simulink model "amila"  (R2013a)
settings: Solver=VariableStepDiscrete  SolverMode=SingleTasking  StartTime=0.0  StopTime=5000  RelTol=1e-3
undefined symbols (not defined in the file or in its folder): gcbh, sfp, xlBlockLoadCallback
libraries: xbsIndex_r4 x4681, dspsigops x32, xps_library x30, casper_library_misc x27, casper_library_delays x2
(part 4 of 43)

== system amila/chan1 ==
  fft_shift : Inport
  sync : Inport  Port=2
  din : Inport  Port=3
  Convert8 : xbsIndex_r4/Convert  gui_display_data_type=Boolean  arith_type=Boolean  n_bits=3  bin_pt=0  float_type=Single  exp_bits=8  fraction_bits=24  quantization=Truncate  overflow=Wrap  en=off  latency=0  dbl_ovrd=off  pipeline=off  block_type=convert
      settings: block_version=11.4
  Logical1 : xbsIndex_r4/Logical  logical_function=OR  inputs=4  en=off  latency=1  precision=Full  arith_type=Unsigned  n_bits=16  bin_pt=0  align_bp=on  dbl_ovrd=off  block_type=logical
  Subsystem6 : Subsystem
  a0p0_1st_shift1 : Subsystem  mask{shift=1, latency=0}
      mask prompts: shift "Number bits to shift right by"; latency "Shift latency"
  bus_create5 : Subsystem  AncestorBlock=casper_library_flow_control/bus_create  mask(bus_create){inputNum=8}
      mask prompts: inputNum "Number of inputs:"
      mask init:
      | bus_create_init(gcb,...
      |     'inputNum', inputNum);
  bus_expand : Subsystem  AncestorBlock=casper_library_flow_control/bus_expand  mask(bus_expand){mode=divisions of equal size, outputNum=4, outputWidth=1, outputBinaryPt=0, outputArithmeticType=0, show_format=off, outputToWorkspace=off, variablePrefix=out, outputToModelAsWell=on}
      mask prompts: outputNum "Number of outputs:"; outputWidth "Output width:"; outputBinaryPt "Output binary point position:"; outputArithmeticType "Output arithmetic type (ufix=0, fix=1, bool=2):"; show_format "Print format string?"; outputToWorkspace "Output to workspace?"; variablePrefix "Variable name prefix:"; outputToModelAsWell "Output to model as well?"
      mask help:
      | Expands a 'bus' made using a bus_create or Xilinx
      | concat block.
      | The input will be divided into the specified number
      | of outputs with the specified arithmetic types.
      | Divisions are made from most significant bit.
      mask init: same as amila/bus_expand6
      settings: AttributesFormatString=4 outputs
      mask TypeOptions mode: divisions of equal size | divisions of arbitrary size
      mask Callback mode: bus_expand_callback();
      mask Callback outputWidth: bus_expand_callback();
      mask Callback outputToWorkspace: bus_expand_callback();
  fft_core : xbsIndex_r4/Black Box  init_code=fft_core2_config  sim_method=Inactive  verbose=off  block_type=blackbox2
  unbus0_2 : Subsystem  AncestorBlock=casper_library_flow_control/bus_expand  mask(bus_expand){mode=divisions of equal size, outputNum=16, outputWidth=18, outputBinaryPt=17, outputArithmeticType=1, show_format=off, outputToWorkspace=off, variablePrefix=out, outputToModelAsWell=on}
      mask prompts: outputNum "Number of outputs:"; outputWidth "Output width:"; outputBinaryPt "Output binary point position:"; outputArithmeticType "Output arithmetic type (ufix=0, fix=1, bool=2):"; show_format "Print format string?"; outputToWorkspace "Output to workspace?"; variablePrefix "Variable name prefix:"; outputToModelAsWell "Output to model as well?"
      mask help:
      | Expands a 'bus' made using a bus_create or Xilinx
      | concat block.
      | The input will be divided into the specified number
      | of outputs with the specified arithmetic types.
      | Divisions are made from most significant bit.
      mask init: same as amila/bus_expand6
      settings: AttributesFormatString=16 outputs
      mask TypeOptions mode: divisions of equal size | divisions of arbitrary size
      mask Callback mode: bus_expand_callback();
      mask Callback outputWidth: bus_expand_callback();
      mask Callback outputToWorkspace: bus_expand_callback();
  sync_out : Outport
  dout : Outport  Port=2
  fft_of : Outport  Port=3
  wires:
  unbus0_2/10(out7) -> Subsystem6/11(In10)
  unbus0_2/12(out5) -> Subsystem6/13(In12)
  unbus0_2/3(out14) -> Subsystem6/4(In3)
  unbus0_2/6(out11) -> Subsystem6/7(In6)
  unbus0_2/16(lsb_out1) -> Subsystem6/17(In16)
  unbus0_2/14(out3) -> Subsystem6/15(In14)
  unbus0_2/5(out12) -> Subsystem6/6(In5)
  unbus0_2/15(out2) -> Subsystem6/16(In15)
  unbus0_2/11(out6) -> Subsystem6/12(In11)
  unbus0_2/9(out8) -> Subsystem6/10(In9)
  unbus0_2/1(msb_out16) -> Subsystem6/2(In1)
  unbus0_2/13(out4) -> Subsystem6/14(In13)
  unbus0_2/2(out15) -> Subsystem6/3(In2)
  unbus0_2/7(out10) -> Subsystem6/8(In7)
  unbus0_2/8(out9) -> Subsystem6/9(In8)
  unbus0_2/4(out13) -> Subsystem6/5(In4)
  sync/1 -> Subsystem6/1(sync)
  bus_create5/1(bus_out) -> dout/1
  fft_shift/1 -> fft_core/1
  a0p0_1st_shift1/1(sync_out) -> fft_core/2
  a0p0_1st_shift1/2(dout1) -> fft_core/3
  a0p0_1st_shift1/3(dout2) -> fft_core/4
  a0p0_1st_shift1/4(dout3) -> fft_core/5
  a0p0_1st_shift1/5(dout4) -> fft_core/6
  a0p0_1st_shift1/6(dout5) -> fft_core/7
  a0p0_1st_shift1/8(dout7) -> fft_core/9
  a0p0_1st_shift1/9(dout8) -> fft_core/10
  a0p0_1st_shift1/10(dout9) -> fft_core/11
  a0p0_1st_shift1/11(dout10) -> fft_core/12
  a0p0_1st_shift1/12(dout11) -> fft_core/13
  a0p0_1st_shift1/13(dout12) -> fft_core/14
  a0p0_1st_shift1/14(dout13) -> fft_core/15
  a0p0_1st_shift1/15(dout14) -> fft_core/16
  a0p0_1st_shift1/16(dout15) -> fft_core/17
  a0p0_1st_shift1/17(dout16) -> fft_core/18
  din/1 -> unbus0_2/1(bus_in)
  Subsystem6/8(Out7) -> a0p0_1st_shift1/8(din7)
  Subsystem6/13(Out12) -> a0p0_1st_shift1/13(din12)
  Subsystem6/11(Out10) -> a0p0_1st_shift1/11(din10)
  Subsystem6/16(Out15) -> a0p0_1st_shift1/16(din15)
  Subsystem6/14(Out13) -> a0p0_1st_shift1/14(din13)
  Subsystem6/10(Out9) -> a0p0_1st_shift1/10(din9)
  Subsystem6/6(Out5) -> a0p0_1st_shift1/6(din5)
  Subsystem6/7(Out6) -> a0p0_1st_shift1/7(din6)
  Subsystem6/2(Out1) -> a0p0_1st_shift1/2(din1)
  Subsystem6/3(Out2) -> a0p0_1st_shift1/3(din2)
  Subsystem6/9(Out8) -> a0p0_1st_shift1/9(din8)
  Subsystem6/1(sync_out) -> a0p0_1st_shift1/1(sync_in)
  Subsystem6/12(Out11) -> a0p0_1st_shift1/12(din11)
  Subsystem6/15(Out14) -> a0p0_1st_shift1/15(din14)
  Subsystem6/17(Out16) -> a0p0_1st_shift1/17(din16)
  Subsystem6/4(Out3) -> a0p0_1st_shift1/4(din3)
  Subsystem6/5(Out4) -> a0p0_1st_shift1/5(din4)
  a0p0_1st_shift1/7(dout6) -> fft_core/8
  bus_expand/3(out2) -> Logical1/3
  bus_expand/2(out3) -> Logical1/2
  bus_expand/4(lsb_out1) -> Logical1/4
  bus_expand/1(msb_out4) -> Logical1/1
  Logical1/1 -> Convert8/1
  Convert8/1 -> fft_of/1
  fft_core/1 -> sync_out/1
  fft_core/5 -> bus_create5/4(in4)
  fft_core/7 -> bus_create5/6(in6)
  fft_core/3 -> bus_create5/2(in2)
  fft_core/4 -> bus_create5/3(in3)
  fft_core/9 -> bus_create5/8(in8)
  fft_core/8 -> bus_create5/7(in7)
  fft_core/2 -> bus_create5/1(in1)
  fft_core/6 -> bus_create5/5(in5)
  fft_core/10 -> bus_expand/1(bus_in)

== system amila/clk_frequency ==
  reg_out : Inport
  amila_clk_frequency_user_data_in : xbsIndex_r4/Gateway Out  inherit_from_input=off  hdl_port=on  timing_constraint=None  locs_specified=off  LOCs={}  UseAsDAC=off  DACChannel='1'  block_type=gatewayout
  convert : xbsIndex_r4/Convert  gui_display_data_type=Fixed-point  arith_type=Unsigned  n_bits=32  bin_pt=0  float_type=Single  exp_bits=8  fraction_bits=24  quantization=Truncate  overflow=Wrap  en=off  latency=0  dbl_ovrd=off  pipeline=off  block_type=convert
  sim_reg_out : Outport
  wires:
  amila_clk_frequency_user_data_in/1 -> sim_reg_out/1
  convert/1 -> amila_clk_frequency_user_data_in/1
  reg_out/1 -> convert/1

== system amila/ct_tvg ==
  note: This TVG should result in each packet containing
      | its frequeny value every 16 bits
      | (assuming the ct is working properly)
  enable : Inport
  sync_in : Inport  Port=2
  din : Inport  Port=3
  Concat{1..4} (4 alike) : xbsIndex_r4/Concat  num_inputs=2  dbl_ovrd=off  block_type=concat
  Concat5 : xbsIndex_r4/Concat  num_inputs=4  dbl_ovrd=off  block_type=concat
  Convert{,1..7} (8 alike) : xbsIndex_r4/Convert  gui_display_data_type=Fixed-point  arith_type=Unsigned  n_bits=channel_bits*2  bin_pt=0  float_type=Single  exp_bits=8  fraction_bits=24  quantization=Truncate  overflow=Wrap  en=off  latency=0  dbl_ovrd=off  pipeline=off  block_type=convert
      settings: block_version=11.4
  Counter1 : xbsIndex_r4/Counter  cnt_type=Free Running  cnt_to=10  operation=Up  start_count=2  cnt_by_val=8  arith_type=Unsigned  n_bits=num_channels_bits  bin_pt=0  load_pin=off  rst=on  en=off  explicit_period=on  period=1  dbl_ovrd=off  use_behavioral_HDL=off  implementation=Fabric  block_type=counter
      settings: block_version=11.4
  Counter2 : xbsIndex_r4/Counter  cnt_type=Free Running  cnt_to=10  operation=Up  start_count=0  cnt_by_val=8  arith_type=Unsigned  n_bits=num_channels_bits  bin_pt=0  load_pin=off  rst=on  en=off  explicit_period=on  period=1  dbl_ovrd=off  use_behavioral_HDL=off  implementation=Fabric  block_type=counter
      settings: block_version=11.4
  Counter3 : xbsIndex_r4/Counter  cnt_type=Free Running  cnt_to=10  operation=Up  start_count=3  cnt_by_val=8  arith_type=Unsigned  n_bits=num_channels_bits  bin_pt=0  load_pin=off  rst=on  en=off  explicit_period=on  period=1  dbl_ovrd=off  use_behavioral_HDL=off  implementation=Fabric  block_type=counter
      settings: block_version=11.4
  Counter4 : xbsIndex_r4/Counter  cnt_type=Free Running  cnt_to=10  operation=Up  start_count=1  cnt_by_val=8  arith_type=Unsigned  n_bits=num_channels_bits  bin_pt=0  load_pin=off  rst=on  en=off  explicit_period=on  period=1  dbl_ovrd=off  use_behavioral_HDL=off  implementation=Fabric  block_type=counter
      settings: block_version=11.4
  Counter5 : xbsIndex_r4/Counter  cnt_type=Free Running  cnt_to=10  operation=Up  start_count=6  cnt_by_val=8  arith_type=Unsigned  n_bits=num_channels_bits  bin_pt=0  load_pin=off  rst=on  en=off  explicit_period=on  period=1  dbl_ovrd=off  use_behavioral_HDL=off  implementation=Fabric  block_type=counter
      settings: block_version=11.4
  Counter6 : xbsIndex_r4/Counter  cnt_type=Free Running  cnt_to=10  operation=Up  start_count=4  cnt_by_val=8  arith_type=Unsigned  n_bits=num_channels_bits  bin_pt=0  load_pin=off  rst=on  en=off  explicit_period=on  period=1  dbl_ovrd=off  use_behavioral_HDL=off  implementation=Fabric  block_type=counter
      settings: block_version=11.4
  Counter7 : xbsIndex_r4/Counter  cnt_type=Free Running  cnt_to=10  operation=Up  start_count=7  cnt_by_val=8  arith_type=Unsigned  n_bits=num_channels_bits  bin_pt=0  load_pin=off  rst=on  en=off  explicit_period=on  period=1  dbl_ovrd=off  use_behavioral_HDL=off  implementation=Fabric  block_type=counter
      settings: block_version=11.4
  Counter8 : xbsIndex_r4/Counter  cnt_type=Free Running  cnt_to=10  operation=Up  start_count=5  cnt_by_val=8  arith_type=Unsigned  n_bits=num_channels_bits  bin_pt=0  load_pin=off  rst=on  en=off  explicit_period=on  period=1  dbl_ovrd=off  use_behavioral_HDL=off  implementation=Fabric  block_type=counter
      settings: block_version=11.4
  Delay : xbsIndex_r4/Delay  rst=off  infoeditControl=Selection of Reset will increase slice count due to use of real FFs and instead of SRLs  en=off  latency=1  dbl_ovrd=off  reg_retiming=off  block_type=delay
      settings: block_version=11.4
  Mux1 : xbsIndex_r4/Mux  inputs=2  en=off  latency=1  precision=Full  arith_type=Unsigned  n_bits=16  bin_pt=14  quantization=Truncate  overflow=Wrap  dbl_ovrd=off  block_type=mux
      settings: block_version=11.4
  Slice{,1..7} (8 alike) : xbsIndex_r4/Slice  nbits=channel_bits  boolean_output=off  mode=Lower Bit Location + Width  bit1=0  base1=MSB of Input  bit0=0  base0=LSB of Input  dbl_ovrd=off  block_type=slice
  sync_out : Outport
  dout : Outport  Port=2
  wires:
  Counter2/1 -> Convert/1
  Counter4/1 -> Convert1/1
  sync_in/1 -> Counter2/1, Delay/1, Counter7/1, Counter5/1, Counter8/1, Counter6/1, Counter3/1, Counter1/1, Counter4/1
  Mux1/1 -> dout/1
  enable/1 -> Mux1/1
  din/1 -> Mux1/2
  Convert/1 -> Slice/1
  Convert1/1 -> Slice1/1
  Delay/1 -> sync_out/1
  Convert2/1 -> Slice2/1
  Convert3/1 -> Slice3/1
  Convert4/1 -> Slice4/1
  Convert5/1 -> Slice5/1
  Convert6/1 -> Slice6/1
  Convert7/1 -> Slice7/1
  Counter1/1 -> Convert2/1
  Counter3/1 -> Convert3/1
  Counter6/1 -> Convert4/1
  Counter8/1 -> Convert5/1
  Counter5/1 -> Convert6/1
  Counter7/1 -> Convert7/1
  Slice/1 -> Concat1/1
  Slice1/1 -> Concat1/2
  Slice2/1 -> Concat2/1
  Slice3/1 -> Concat2/2
  Slice4/1 -> Concat3/1
  Slice5/1 -> Concat3/2
  Slice6/1 -> Concat4/1
  Slice7/1 -> Concat4/2
  Concat2/1 -> Concat5/2
  Concat3/1 -> Concat5/3
  Concat1/1 -> Concat5/1
  Concat4/1 -> Concat5/4
  Concat5/1 -> Mux1/3

== system amila/ct_tvg1 ==
  note: This TVG should result in each packet containing
      | its frequeny value every 16 bits
      | (assuming the ct is working properly)
  enable : Inport
  sync_in : Inport  Port=2
  din : Inport  Port=3
  Concat{1..4} (4 alike) : xbsIndex_r4/Concat  num_inputs=2  dbl_ovrd=off  block_type=concat
  Concat5 : xbsIndex_r4/Concat  num_inputs=4  dbl_ovrd=off  block_type=concat
  Convert{,1..7} (8 alike) : xbsIndex_r4/Convert  gui_display_data_type=Fixed-point  arith_type=Unsigned  n_bits=channel_bits*2  bin_pt=0  float_type=Single  exp_bits=8  fraction_bits=24  quantization=Truncate  overflow=Wrap  en=off  latency=0  dbl_ovrd=off  pipeline=off  block_type=convert
      settings: block_version=11.4
  Counter1 : xbsIndex_r4/Counter  cnt_type=Free Running  cnt_to=10  operation=Up  start_count=2  cnt_by_val=8  arith_type=Unsigned  n_bits=num_channels_bits  bin_pt=0  load_pin=off  rst=on  en=off  explicit_period=on  period=1  dbl_ovrd=off  use_behavioral_HDL=off  implementation=Fabric  block_type=counter
      settings: block_version=11.4
  Counter2 : xbsIndex_r4/Counter  cnt_type=Free Running  cnt_to=10  operation=Up  start_count=0  cnt_by_val=8  arith_type=Unsigned  n_bits=num_channels_bits  bin_pt=0  load_pin=off  rst=on  en=off  explicit_period=on  period=1  dbl_ovrd=off  use_behavioral_HDL=off  implementation=Fabric  block_type=counter
      settings: block_version=11.4
  Counter3 : xbsIndex_r4/Counter  cnt_type=Free Running  cnt_to=10  operation=Up  start_count=3  cnt_by_val=8  arith_type=Unsigned  n_bits=num_channels_bits  bin_pt=0  load_pin=off  rst=on  en=off  explicit_period=on  period=1  dbl_ovrd=off  use_behavioral_HDL=off  implementation=Fabric  block_type=counter
      settings: block_version=11.4
  Counter4 : xbsIndex_r4/Counter  cnt_type=Free Running  cnt_to=10  operation=Up  start_count=1  cnt_by_val=8  arith_type=Unsigned  n_bits=num_channels_bits  bin_pt=0  load_pin=off  rst=on  en=off  explicit_period=on  period=1  dbl_ovrd=off  use_behavioral_HDL=off  implementation=Fabric  block_type=counter
      settings: block_version=11.4
  Counter5 : xbsIndex_r4/Counter  cnt_type=Free Running  cnt_to=10  operation=Up  start_count=6  cnt_by_val=8  arith_type=Unsigned  n_bits=num_channels_bits  bin_pt=0  load_pin=off  rst=on  en=off  explicit_period=on  period=1  dbl_ovrd=off  use_behavioral_HDL=off  implementation=Fabric  block_type=counter
      settings: block_version=11.4
  Counter6 : xbsIndex_r4/Counter  cnt_type=Free Running  cnt_to=10  operation=Up  start_count=4  cnt_by_val=8  arith_type=Unsigned  n_bits=num_channels_bits  bin_pt=0  load_pin=off  rst=on  en=off  explicit_period=on  period=1  dbl_ovrd=off  use_behavioral_HDL=off  implementation=Fabric  block_type=counter
      settings: block_version=11.4
  Counter7 : xbsIndex_r4/Counter  cnt_type=Free Running  cnt_to=10  operation=Up  start_count=7  cnt_by_val=8  arith_type=Unsigned  n_bits=num_channels_bits  bin_pt=0  load_pin=off  rst=on  en=off  explicit_period=on  period=1  dbl_ovrd=off  use_behavioral_HDL=off  implementation=Fabric  block_type=counter
      settings: block_version=11.4
  Counter8 : xbsIndex_r4/Counter  cnt_type=Free Running  cnt_to=10  operation=Up  start_count=5  cnt_by_val=8  arith_type=Unsigned  n_bits=num_channels_bits  bin_pt=0  load_pin=off  rst=on  en=off  explicit_period=on  period=1  dbl_ovrd=off  use_behavioral_HDL=off  implementation=Fabric  block_type=counter
      settings: block_version=11.4
  Delay : xbsIndex_r4/Delay  rst=off  infoeditControl=Selection of Reset will increase slice count due to use of real FFs and instead of SRLs  en=off  latency=1  dbl_ovrd=off  reg_retiming=off  block_type=delay
      settings: block_version=11.4
  Mux1 : xbsIndex_r4/Mux  inputs=2  en=off  latency=1  precision=Full  arith_type=Unsigned  n_bits=16  bin_pt=14  quantization=Truncate  overflow=Wrap  dbl_ovrd=off  block_type=mux
      settings: block_version=11.4
  Slice{,1..7} (8 alike) : xbsIndex_r4/Slice  nbits=channel_bits  boolean_output=off  mode=Lower Bit Location + Width  bit1=0  base1=MSB of Input  bit0=0  base0=LSB of Input  dbl_ovrd=off  block_type=slice
  sync_out : Outport
  dout : Outport  Port=2
  wires:
  Concat5/1 -> Mux1/3
  Concat4/1 -> Concat5/4
  Concat1/1 -> Concat5/1
  Concat3/1 -> Concat5/3
  Concat2/1 -> Concat5/2
  Slice7/1 -> Concat4/2
  Slice6/1 -> Concat4/1
  Slice5/1 -> Concat3/2
  Slice4/1 -> Concat3/1
  Slice3/1 -> Concat2/2
  Slice2/1 -> Concat2/1
  Slice1/1 -> Concat1/2
  Slice/1 -> Concat1/1
  Counter7/1 -> Convert7/1
  Counter5/1 -> Convert6/1
  Counter8/1 -> Convert5/1
  Counter6/1 -> Convert4/1
  Counter3/1 -> Convert3/1
  Counter1/1 -> Convert2/1
  Convert7/1 -> Slice7/1
  Convert6/1 -> Slice6/1
  Convert5/1 -> Slice5/1
  Convert4/1 -> Slice4/1
  Convert3/1 -> Slice3/1
  Convert2/1 -> Slice2/1
  Delay/1 -> sync_out/1
  Convert1/1 -> Slice1/1
  Convert/1 -> Slice/1
  din/1 -> Mux1/2
  enable/1 -> Mux1/1
  Mux1/1 -> dout/1
  sync_in/1 -> Counter4/1, Counter1/1, Counter3/1, Counter6/1, Counter8/1, Counter5/1, Counter7/1, Delay/1, Counter2/1
  Counter4/1 -> Convert1/1
  Counter2/1 -> Convert/1

== system amila/delay_0 ==
  sync : Inport
  delay : Inport  Port=2
  din : Inport  Port=3
  Delay14 : xbsIndex_r4/Delay  rst=off  infoeditControl=Selection of Reset will increase slice count due to use of real FFs and instead of SRLs  en=off  latency=1  dbl_ovrd=off  reg_retiming=off  block_type=delay
      settings: block_version=11.4
  Subsystem3 : Subsystem
  bus_create5 : Subsystem  AncestorBlock=casper_library_flow_control/bus_create  mask(bus_create){inputNum=16}
      mask prompts: inputNum "Number of inputs:"
      mask init:
      | bus_create_init(gcb,...
      |     'inputNum', inputNum);
  delay_core : xbsIndex_r4/Black Box  init_code=delay_core_config  sim_method=Inactive  verbose=off  block_type=blackbox2
      settings: block_version=11.4
  pipeline10 : Subsystem
  unbus0_3 : Subsystem  AncestorBlock=casper_library_flow_control/bus_expand  mask(bus_expand){mode=divisions of equal size, outputNum=16, outputWidth=8, outputBinaryPt=0, outputArithmeticType=0, show_format=off, outputToWorkspace=off, variablePrefix=out, outputToModelAsWell=on}
      mask prompts: outputNum "Number of outputs:"; outputWidth "Output width:"; outputBinaryPt "Output binary point position:"; outputArithmeticType "Output arithmetic type (ufix=0, fix=1, bool=2):"; show_format "Print format string?"; outputToWorkspace "Output to workspace?"; variablePrefix "Variable name prefix:"; outputToModelAsWell "Output to model as well?"
      mask help:
      | Expands a 'bus' made using a bus_create or Xilinx
      | concat block.
      | The input will be divided into the specified number
      | of outputs with the specified arithmetic types.
      | Divisions are made from most significant bit.
      mask init: same as amila/bus_expand6
      settings: AttributesFormatString=16 outputs
      mask TypeOptions mode: divisions of equal size | divisions of arbitrary size
      mask Callback mode: bus_expand_callback();
      mask Callback outputWidth: bus_expand_callback();
      mask Callback outputToWorkspace: bus_expand_callback();
  sync_out : Outport
  dout : Outport  Port=2
  wires:
  bus_create5/1(bus_out) -> dout/1
  Subsystem3/3(Out2) -> bus_create5/2(in2)
  Subsystem3/10(Out9) -> bus_create5/9(in9)
  Subsystem3/14(Out13) -> bus_create5/13(in13)
  Subsystem3/15(Out14) -> bus_create5/14(in14)
  Subsystem3/7(Out6) -> bus_create5/6(in6)
  Subsystem3/13(Out12) -> bus_create5/12(in12)
  Subsystem3/12(Out11) -> bus_create5/11(in11)
  Subsystem3/9(Out8) -> bus_create5/8(in8)
  Subsystem3/8(Out7) -> bus_create5/7(in7)
  Subsystem3/16(Out15) -> bus_create5/15(in15)
  Subsystem3/17(Out16) -> bus_create5/16(in16)
  Subsystem3/4(Out3) -> bus_create5/3(in3)
  Subsystem3/11(Out10) -> bus_create5/10(in10)
  Subsystem3/5(Out4) -> bus_create5/4(in4)
  Subsystem3/2(Out1) -> bus_create5/1(in1)
  Subsystem3/6(Out5) -> bus_create5/5(in5)
  delay_core/7 -> Subsystem3/7(In6)
  delay_core/6 -> Subsystem3/6(In5)
  delay_core/14 -> Subsystem3/14(In13)
  delay_core/13 -> Subsystem3/13(In12)
  delay_core/9 -> Subsystem3/9(In8)
  delay_core/11 -> Subsystem3/11(In10)
  delay_core/1 -> Subsystem3/1(sync)
  delay_core/15 -> Subsystem3/15(In14)
  delay_core/2 -> Subsystem3/2(In1)
  delay_core/17 -> Subsystem3/17(In16)
  delay_core/4 -> Subsystem3/4(In3)
  delay_core/10 -> Subsystem3/10(In9)
  delay_core/12 -> Subsystem3/12(In11)
  delay_core/5 -> Subsystem3/5(In4)
  delay_core/8 -> Subsystem3/8(In7)
  delay_core/3 -> Subsystem3/3(In2)
  delay_core/16 -> Subsystem3/16(In15)
  unbus0_3/16(lsb_out1) -> pipeline10/16(In16)
  unbus0_3/15(out2) -> pipeline10/15(In15)
  unbus0_3/14(out3) -> pipeline10/14(In14)
  unbus0_3/13(out4) -> pipeline10/13(In13)
  unbus0_3/12(out5) -> pipeline10/12(In12)
  unbus0_3/11(out6) -> pipeline10/11(In11)
  unbus0_3/10(out7) -> pipeline10/10(In10)
  unbus0_3/9(out8) -> pipeline10/9(In9)
  unbus0_3/8(out9) -> pipeline10/8(In8)
  unbus0_3/7(out10) -> pipeline10/7(In7)
  unbus0_3/6(out11) -> pipeline10/6(In6)
  unbus0_3/5(out12) -> pipeline10/5(In5)
  unbus0_3/4(out13) -> pipeline10/4(In4)
  unbus0_3/3(out14) -> pipeline10/3(In3)
  unbus0_3/2(out15) -> pipeline10/2(In2)
  unbus0_3/1(msb_out16) -> pipeline10/1(In1)
  sync/1 -> Delay14/1
  Delay14/1 -> delay_core/3, delay_core/1
  din/1 -> unbus0_3/1(bus_in)
  delay/1 -> delay_core/2
  Subsystem3/1(sync_out) -> sync_out/1
  pipeline10/16(Out16) -> delay_core/19
  pipeline10/15(Out15) -> delay_core/18
  pipeline10/14(Out14) -> delay_core/17
  pipeline10/13(Out13) -> delay_core/16
  pipeline10/12(Out12) -> delay_core/15
  pipeline10/11(Out11) -> delay_core/14
  pipeline10/10(Out10) -> delay_core/13
  pipeline10/9(Out9) -> delay_core/12
  pipeline10/8(Out8) -> delay_core/11
  pipeline10/7(Out7) -> delay_core/10
  pipeline10/6(Out6) -> delay_core/9
  pipeline10/5(Out5) -> delay_core/8
  pipeline10/4(Out4) -> delay_core/7
  pipeline10/3(Out3) -> delay_core/6
  pipeline10/2(Out2) -> delay_core/5
  pipeline10/1(Out1) -> delay_core/4

== system amila/delay_1 ==
  sync : Inport
  delay : Inport  Port=2
  din : Inport  Port=3
  Delay14 : xbsIndex_r4/Delay  rst=off  infoeditControl=Selection of Reset will increase slice count due to use of real FFs and instead of SRLs  en=off  latency=1  dbl_ovrd=off  reg_retiming=off  block_type=delay
      settings: block_version=11.4
  Subsystem3 : Subsystem
  bus_create5 : Subsystem  AncestorBlock=casper_library_flow_control/bus_create  mask(bus_create){inputNum=16}
      mask prompts: inputNum "Number of inputs:"
      mask init:
      | bus_create_init(gcb,...
      |     'inputNum', inputNum);
  delay_core : xbsIndex_r4/Black Box  init_code=delay_core_config  sim_method=Inactive  verbose=off  block_type=blackbox2
      settings: block_version=11.4
  pipeline10 : Subsystem
  unbus0_3 : Subsystem  AncestorBlock=casper_library_flow_control/bus_expand  mask(bus_expand){mode=divisions of equal size, outputNum=16, outputWidth=8, outputBinaryPt=0, outputArithmeticType=0, show_format=off, outputToWorkspace=off, variablePrefix=out, outputToModelAsWell=on}
      mask prompts: outputNum "Number of outputs:"; outputWidth "Output width:"; outputBinaryPt "Output binary point position:"; outputArithmeticType "Output arithmetic type (ufix=0, fix=1, bool=2):"; show_format "Print format string?"; outputToWorkspace "Output to workspace?"; variablePrefix "Variable name prefix:"; outputToModelAsWell "Output to model as well?"
      mask help:
      | Expands a 'bus' made using a bus_create or Xilinx
      | concat block.
      | The input will be divided into the specified number
      | of outputs with the specified arithmetic types.
      | Divisions are made from most significant bit.
      mask init: same as amila/bus_expand6
      settings: AttributesFormatString=16 outputs
      mask TypeOptions mode: divisions of equal size | divisions of arbitrary size
      mask Callback mode: bus_expand_callback();
      mask Callback outputWidth: bus_expand_callback();
      mask Callback outputToWorkspace: bus_expand_callback();
  sync_out : Outport
  dout : Outport  Port=2
  wires:
  pipeline10/1(Out1) -> delay_core/4
  pipeline10/2(Out2) -> delay_core/5
  pipeline10/3(Out3) -> delay_core/6
  pipeline10/4(Out4) -> delay_core/7
  pipeline10/5(Out5) -> delay_core/8
  pipeline10/6(Out6) -> delay_core/9
  pipeline10/7(Out7) -> delay_core/10
  pipeline10/8(Out8) -> delay_core/11
  pipeline10/9(Out9) -> delay_core/12
  pipeline10/10(Out10) -> delay_core/13
  pipeline10/11(Out11) -> delay_core/14
  pipeline10/12(Out12) -> delay_core/15
  pipeline10/13(Out13) -> delay_core/16
  pipeline10/14(Out14) -> delay_core/17
  pipeline10/15(Out15) -> delay_core/18
  pipeline10/16(Out16) -> delay_core/19
  Subsystem3/1(sync_out) -> sync_out/1
  delay/1 -> delay_core/2
  din/1 -> unbus0_3/1(bus_in)
  Delay14/1 -> delay_core/3, delay_core/1
  sync/1 -> Delay14/1
  unbus0_3/1(msb_out16) -> pipeline10/1(In1)
  unbus0_3/2(out15) -> pipeline10/2(In2)
  unbus0_3/3(out14) -> pipeline10/3(In3)
  unbus0_3/4(out13) -> pipeline10/4(In4)
  unbus0_3/5(out12) -> pipeline10/5(In5)
  unbus0_3/6(out11) -> pipeline10/6(In6)
  unbus0_3/7(out10) -> pipeline10/7(In7)
  unbus0_3/8(out9) -> pipeline10/8(In8)
  unbus0_3/9(out8) -> pipeline10/9(In9)
  unbus0_3/10(out7) -> pipeline10/10(In10)
  unbus0_3/11(out6) -> pipeline10/11(In11)
  unbus0_3/12(out5) -> pipeline10/12(In12)
  unbus0_3/13(out4) -> pipeline10/13(In13)
  unbus0_3/14(out3) -> pipeline10/14(In14)
  unbus0_3/15(out2) -> pipeline10/15(In15)
  unbus0_3/16(lsb_out1) -> pipeline10/16(In16)
  delay_core/16 -> Subsystem3/16(In15)
  delay_core/3 -> Subsystem3/3(In2)
  delay_core/8 -> Subsystem3/8(In7)
  delay_core/5 -> Subsystem3/5(In4)
  delay_core/12 -> Subsystem3/12(In11)
  delay_core/10 -> Subsystem3/10(In9)
  delay_core/4 -> Subsystem3/4(In3)
  delay_core/17 -> Subsystem3/17(In16)
  delay_core/2 -> Subsystem3/2(In1)
  delay_core/15 -> Subsystem3/15(In14)
  delay_core/1 -> Subsystem3/1(sync)
  delay_core/11 -> Subsystem3/11(In10)
  delay_core/9 -> Subsystem3/9(In8)
  delay_core/13 -> Subsystem3/13(In12)
  delay_core/14 -> Subsystem3/14(In13)
  delay_core/6 -> Subsystem3/6(In5)
  delay_core/7 -> Subsystem3/7(In6)
  Subsystem3/6(Out5) -> bus_create5/5(in5)
  Subsystem3/2(Out1) -> bus_create5/1(in1)
  Subsystem3/5(Out4) -> bus_create5/4(in4)
  Subsystem3/11(Out10) -> bus_create5/10(in10)
  Subsystem3/4(Out3) -> bus_create5/3(in3)
  Subsystem3/17(Out16) -> bus_create5/16(in16)
  Subsystem3/16(Out15) -> bus_create5/15(in15)
  Subsystem3/8(Out7) -> bus_create5/7(in7)
  Subsystem3/9(Out8) -> bus_create5/8(in8)
  Subsystem3/12(Out11) -> bus_create5/11(in11)
  Subsystem3/13(Out12) -> bus_create5/12(in12)
  Subsystem3/7(Out6) -> bus_create5/6(in6)
  Subsystem3/15(Out14) -> bus_create5/14(in14)
  Subsystem3/14(Out13) -> bus_create5/13(in13)
  Subsystem3/10(Out9) -> bus_create5/9(in9)
  Subsystem3/3(Out2) -> bus_create5/2(in2)
  bus_create5/1(bus_out) -> dout/1

== system amila/edge_detect ==
  in : Inport
  Delay : xbsIndex_r4/Delay  rst=off  infoeditControl=Selection of Reset will increase slice count due to use of real FFs and instead of SRLs  en=off  latency=1  dbl_ovrd=off  reg_retiming=off  block_type=delay
      settings: xl_area=[0, 0, 0, 0, 0, 0, 0]
  Inverter : xbsIndex_r4/Inverter  en=off  latency=0  dbl_ovrd=off  block_type=inv
      settings: xl_area=[0, 0, 0, 0, 0, 0, 0]
  edge_op : xbsIndex_r4/Logical  logical_function=AND  inputs=2  en=off  latency=0  precision=Full  arith_type=Unsigned  n_bits=8  bin_pt=2  align_bp=on  dbl_ovrd=off  block_type=logical
      settings: xl_area=[0, 0, 0, 0, 0, 0, 0]
  out : Outport
  wires:
  Inverter/1 -> edge_op/1
  edge_op/1 -> out/1
  in/1 -> Inverter/1, Delay/1
  Delay/1 -> edge_op/2

== system amila/edge_detect1 ==
  in : Inport
  Delay : xbsIndex_r4/Delay  rst=off  infoeditControl=Selection of Reset will increase slice count due to use of real FFs and instead of SRLs  en=off  latency=1  dbl_ovrd=off  reg_retiming=off  block_type=delay
      settings: xl_area=[0, 0, 0, 0, 0, 0, 0]
  Inverter : xbsIndex_r4/Inverter  en=off  latency=0  dbl_ovrd=off  block_type=inv
      settings: xl_area=[0, 0, 0, 0, 0, 0, 0]
  edge_op : xbsIndex_r4/Logical  logical_function=NOR  inputs=2  en=off  latency=0  precision=Full  arith_type=Unsigned  n_bits=8  bin_pt=2  align_bp=on  dbl_ovrd=off  block_type=logical
      settings: xl_area=[0, 0, 0, 0, 0, 0, 0]
  out : Outport
  wires:
  Inverter/1 -> edge_op/1
  edge_op/1 -> out/1
  in/1 -> Inverter/1, Delay/1
  Delay/1 -> edge_op/2

== system amila/feng0_adc_acc_len ==
  sim_1 : Inport
  amila_feng0_adc_acc_len_user_data_out : xbsIndex_r4/Gateway In  gui_display_data_type=Fixed-point  arith_type=Unsigned  n_bits=32  bin_pt=0  preci_type=Single  exp_width=8  frac_width=24  quantization="Round  (unbiased: +/- Inf)"  overflow=Saturate  period=1  dbl_ovrd=off  timing_constraint=None  locs_specified=off  LOCs={}  UseAsADC=off  ADCChannel='1'  inherit_from_input=off  hdl_port=on  block_type=gatewayin
  io_delay : xbsIndex_r4/Delay  rst=off  infoeditControl=Selection of Reset will increase slice count due to use of real FFs and instead of SRLs  en=off  latency=0  dbl_ovrd=off  reg_retiming=on  block_type=delay
  reint1 : xbsIndex_r4/Reinterpret  force_arith_type=on  arith_type=Unsigned  force_bin_pt=on  bin_pt=0  block_type=reinterpret
  slice_reg : xbsIndex_r4/Slice  nbits=32  boolean_output=off  mode=Lower Bit Location + Width  bit1=0  base1=MSB of Input  bit0=0  base0=LSB of Input  dbl_ovrd=off  block_type=slice
  in_reg : Outport
  wires:
  amila_feng0_adc_acc_len_user_data_out/1 -> io_delay/1
  sim_1/1 -> amila_feng0_adc_acc_len_user_data_out/1
  io_delay/1 -> slice_reg/1
  slice_reg/1 -> reint1/1
  reint1/1 -> in_reg/1

== system amila/feng0_adc_sum_sq0 ==
  reg_out : Inport
  amila_feng0_adc_sum_sq0_user_data_in : xbsIndex_r4/Gateway Out  inherit_from_input=off  hdl_port=on  timing_constraint=None  locs_specified=off  LOCs={}  UseAsDAC=off  DACChannel='1'  block_type=gatewayout
  convert : xbsIndex_r4/Convert  gui_display_data_type=Fixed-point  arith_type=Unsigned  n_bits=32  bin_pt=0  float_type=Single  exp_bits=8  fraction_bits=24  quantization=Truncate  overflow=Wrap  en=off  latency=0  dbl_ovrd=off  pipeline=off  block_type=convert
  sim_reg_out : Outport
  wires:
  amila_feng0_adc_sum_sq0_user_data_in/1 -> sim_reg_out/1
  convert/1 -> amila_feng0_adc_sum_sq0_user_data_in/1
  reg_out/1 -> convert/1

== system amila/feng0_adc_sum_sq1 ==
  reg_out : Inport
  amila_feng0_adc_sum_sq1_user_data_in : xbsIndex_r4/Gateway Out  inherit_from_input=off  hdl_port=on  timing_constraint=None  locs_specified=off  LOCs={}  UseAsDAC=off  DACChannel='1'  block_type=gatewayout
  convert : xbsIndex_r4/Convert  gui_display_data_type=Fixed-point  arith_type=Unsigned  n_bits=32  bin_pt=0  float_type=Single  exp_bits=8  fraction_bits=24  quantization=Truncate  overflow=Wrap  en=off  latency=0  dbl_ovrd=off  pipeline=off  block_type=convert
  sim_reg_out : Outport
  wires:
  amila_feng0_adc_sum_sq1_user_data_in/1 -> sim_reg_out/1
  convert/1 -> amila_feng0_adc_sum_sq1_user_data_in/1
  reg_out/1 -> convert/1

== system amila/feng0_ant_id ==
  sim_1 : Inport
  amila_feng0_ant_id_user_data_out : xbsIndex_r4/Gateway In  gui_display_data_type=Fixed-point  arith_type=Unsigned  n_bits=32  bin_pt=0  preci_type=Single  exp_width=8  frac_width=24  quantization="Round  (unbiased: +/- Inf)"  overflow=Saturate  period=1  dbl_ovrd=off  timing_constraint=None  locs_specified=off  LOCs={}  UseAsADC=off  ADCChannel='1'  inherit_from_input=off  hdl_port=on  block_type=gatewayin
  io_delay : xbsIndex_r4/Delay  rst=off  infoeditControl=Selection of Reset will increase slice count due to use of real FFs and instead of SRLs  en=off  latency=0  dbl_ovrd=off  reg_retiming=on  block_type=delay
  reint1 : xbsIndex_r4/Reinterpret  force_arith_type=on  arith_type=Unsigned  force_bin_pt=on  bin_pt=0  block_type=reinterpret
  slice_reg : xbsIndex_r4/Slice  nbits=32  boolean_output=off  mode=Lower Bit Location + Width  bit1=0  base1=MSB of Input  bit0=0  base0=LSB of Input  dbl_ovrd=off  block_type=slice
  in_reg : Outport
  wires:
  amila_feng0_ant_id_user_data_out/1 -> io_delay/1
  sim_1/1 -> amila_feng0_ant_id_user_data_out/1
  io_delay/1 -> slice_reg/1
  slice_reg/1 -> reint1/1
  reint1/1 -> in_reg/1

== system amila/feng0_auto_acc_len ==
  sim_1 : Inport
  amila_feng0_auto_acc_len_user_data_out : xbsIndex_r4/Gateway In  gui_display_data_type=Fixed-point  arith_type=Unsigned  n_bits=32  bin_pt=0  preci_type=Single  exp_width=8  frac_width=24  quantization="Round  (unbiased: +/- Inf)"  overflow=Saturate  period=1  dbl_ovrd=off  timing_constraint=None  locs_specified=off  LOCs={}  UseAsADC=off  ADCChannel='1'  inherit_from_input=off  hdl_port=on  block_type=gatewayin
  io_delay : xbsIndex_r4/Delay  rst=off  infoeditControl=Selection of Reset will increase slice count due to use of real FFs and instead of SRLs  en=off  latency=0  dbl_ovrd=off  reg_retiming=on  block_type=delay
  reint1 : xbsIndex_r4/Reinterpret  force_arith_type=on  arith_type=Unsigned  force_bin_pt=on  bin_pt=0  block_type=reinterpret
  slice_reg : xbsIndex_r4/Slice  nbits=32  boolean_output=off  mode=Lower Bit Location + Width  bit1=0  base1=MSB of Input  bit0=0  base0=LSB of Input  dbl_ovrd=off  block_type=slice
  in_reg : Outport
  wires:
  amila_feng0_auto_acc_len_user_data_out/1 -> io_delay/1
  sim_1/1 -> amila_feng0_auto_acc_len_user_data_out/1
  io_delay/1 -> slice_reg/1
  slice_reg/1 -> reint1/1
  reint1/1 -> in_reg/1

== system amila/feng0_auto_snap ==
  din0 : Inport
  din1 : Inport  Port=2
  din2 : Inport  Port=3
  din3 : Inport  Port=4
  din4 : Inport  Port=5
  din5 : Inport  Port=6
  din6 : Inport  Port=7
  din7 : Inport  Port=8
  we : Inport  Port=9
  trig : Inport  Port=10
  0 : Subsystem  Tag=casper:snapshot  AncestorBlock=casper_library_scopes/snapshot  mask(snapshot){storage=bram, dram_dimm=1, dram_clock=200, nsamples=8, data_width=128, offset=off, circap=off, value=off, use_dsp48=off}
      mask prompts: storage "Storage medium"; dram_dimm "DRAM dimm"; dram_clock "DRAM clock rate"; nsamples "Number of Samples (2^?)"; data_width "Data width"; offset "Start delay support"; circap "Circular capture support"; value "Extra value capture support"; use_dsp48 "Use DSP48s to implement counters"
      mask help:
      | Standard snap block, but with the following optional extras;
      |  1) Optionally delay the fabric trigger by a user-specified number of valids.
      |  2) Capture continuously after a trigger until a stop pulse is received. Data is captured into BRAM continuously, with old data being overwritten until a stop command is received. Then stop capturing when memory is filled. This enables you to get some data before and some data after the stop pulse. Use the 'tr_en_cnt' register to determine where you are in your vector. 'Addr' register's MSb now indicates 'busy capturing'.
      |  3) Optionally capture a value on an input port to a register at the same time as the first data sample.
      |  4) Implement counters using DSP48Es to save resources.
      mask init: same as amila/feng0_quant_snap
      mask TypeOptions storage: bram | dram
      mask Callback storage: snapshot_callback();
      mask TypeOptions dram_dimm: 1 | 2 | 3 | 4
      mask TypeOptions dram_clock: 200 | 250 | 266 | 300 | 333
      mask TypeOptions data_width: 8 | 16 | 32 | 64 | 128
  1 : Subsystem  Tag=casper:snapshot  AncestorBlock=casper_library_scopes/snapshot  mask(snapshot){storage=bram, dram_dimm=1, dram_clock=200, nsamples=8, data_width=128, offset=off, circap=off, value=off, use_dsp48=off}
      mask prompts: storage "Storage medium"; dram_dimm "DRAM dimm"; dram_clock "DRAM clock rate"; nsamples "Number of Samples (2^?)"; data_width "Data width"; offset "Start delay support"; circap "Circular capture support"; value "Extra value capture support"; use_dsp48 "Use DSP48s to implement counters"
      mask help:
      | Standard snap block, but with the following optional extras;
      |  1) Optionally delay the fabric trigger by a user-specified number of valids.
      |  2) Capture continuously after a trigger until a stop pulse is received. Data is captured into BRAM continuously, with old data being overwritten until a stop command is received. Then stop capturing when memory is filled. This enables you to get some data before and some data after the stop pulse. Use the 'tr_en_cnt' register to determine where you are in your vector. 'Addr' register's MSb now indicates 'busy capturing'.
      |  3) Optionally capture a value on an input port to a register at the same time as the first data sample.
      |  4) Implement counters using DSP48Es to save resources.
      mask init: same as amila/feng0_quant_snap
      mask TypeOptions storage: bram | dram
      mask Callback storage: snapshot_callback();
      mask TypeOptions dram_dimm: 1 | 2 | 3 | 4
      mask TypeOptions dram_clock: 200 | 250 | 266 | 300 | 333
      mask TypeOptions data_width: 8 | 16 | 32 | 64 | 128
  2 : Subsystem  Tag=casper:snapshot  AncestorBlock=casper_library_scopes/snapshot  mask(snapshot){storage=bram, dram_dimm=1, dram_clock=200, nsamples=8, data_width=128, offset=off, circap=off, value=off, use_dsp48=off}
      mask prompts: storage "Storage medium"; dram_dimm "DRAM dimm"; dram_clock "DRAM clock rate"; nsamples "Number of Samples (2^?)"; data_width "Data width"; offset "Start delay support"; circap "Circular capture support"; value "Extra value capture support"; use_dsp48 "Use DSP48s to implement counters"
      mask help:
      | Standard snap block, but with the following optional extras;
      |  1) Optionally delay the fabric trigger by a user-specified number of valids.
      |  2) Capture continuously after a trigger until a stop pulse is received. Data is captured into BRAM continuously, with old data being overwritten until a stop command is received. Then stop capturing when memory is filled. This enables you to get some data before and some data after the stop pulse. Use the 'tr_en_cnt' register to determine where you are in your vector. 'Addr' register's MSb now indicates 'busy capturing'.
      |  3) Optionally capture a value on an input port to a register at the same time as the first data sample.
      |  4) Implement counters using DSP48Es to save resources.
      mask init: same as amila/feng0_quant_snap
      mask TypeOptions storage: bram | dram
      mask Callback storage: snapshot_callback();
      mask TypeOptions dram_dimm: 1 | 2 | 3 | 4
      mask TypeOptions dram_clock: 200 | 250 | 266 | 300 | 333
      mask TypeOptions data_width: 8 | 16 | 32 | 64 | 128
  Convert{,1..7} (8 alike) : xbsIndex_r4/Convert  gui_display_data_type=Fixed-point  arith_type="Signed  (2's comp)"  n_bits=48  bin_pt=0  float_type=Single  exp_bits=8  fraction_bits=24  quantization=Truncate  overflow=Wrap  en=off  latency=0  dbl_ovrd=off  pipeline=off  block_type=convert
      settings: block_version=11.4
  bus_create : Subsystem  AncestorBlock=casper_library_flow_control/bus_create  mask(bus_create){inputNum=8}
      mask prompts: inputNum "Number of inputs:"
      mask init:
      | bus_create_init(gcb,...
      |     'inputNum', inputNum);
  bus_expand : Subsystem  AncestorBlock=casper_library_flow_control/bus_expand  mask(bus_expand){mode=divisions of equal size, outputNum=3, outputWidth=128, outputBinaryPt=0, outputArithmeticType=0, show_format=off, outputToWorkspace=off, variablePrefix=out, outputToModelAsWell=on}
      mask prompts: outputNum "Number of outputs:"; outputWidth "Output width:"; outputBinaryPt "Output binary point position:"; outputArithmeticType "Output arithmetic type (ufix=0, fix=1, bool=2):"; show_format "Print format string?"; outputToWorkspace "Output to workspace?"; variablePrefix "Variable name prefix:"; outputToModelAsWell "Output to model as well?"
      mask help:
      | Expands a 'bus' made using a bus_create or Xilinx
      | concat block.
      | The input will be divided into the specified number
      | of outputs with the specified arithmetic types.
      | Divisions are made from most significant bit.
      mask init: same as amila/bus_expand6
      settings: AttributesFormatString=3 outputs
      mask TypeOptions mode: divisions of equal size | divisions of arbitrary size
      mask Callback mode: bus_expand_callback();
      mask Callback outputWidth: bus_expand_callback();
      mask Callback outputToWorkspace: bus_expand_callback();
  reg{1..14} (14 alike) : xbsIndex_r4/Delay  rst=off  infoeditControl=Selection of Reset will increase slice count due to use of real FFs and instead of SRLs  en=off  latency=1  dbl_ovrd=off  reg_retiming=off  block_type=delay
  wires:
  bus_expand/2(out2) -> 1/1(din)
  bus_expand/3(lsb_out1) -> 2/1(din)
  bus_expand/1(msb_out3) -> 0/1(din)
  bus_create/1(bus_out) -> bus_expand/1(bus_in)
  [trig] -> reg13/1
  [we] -> reg14/1
  reg13/1 -> 2/3(trig)
  reg14/1 -> 2/2(we)
  [trig] -> reg11/1
  [we] -> reg12/1
  reg11/1 -> 1/3(trig)
  reg12/1 -> 1/2(we)
  [trig] -> reg10/1
  [we] -> reg8/1
  reg10/1 -> 0/3(trig)
  reg8/1 -> 0/2(we)
  Convert7/1 -> bus_create/8(in8)
  Convert6/1 -> bus_create/7(in7)
  Convert5/1 -> bus_create/6(in6)
  Convert4/1 -> bus_create/5(in5)
  Convert3/1 -> bus_create/4(in4)
  Convert2/1 -> bus_create/3(in3)
  Convert1/1 -> bus_create/2(in2)
  Convert/1 -> bus_create/1(in1)
  reg5/1 -> Convert7/1
  reg6/1 -> Convert6/1
  reg4/1 -> Convert5/1
  reg7/1 -> Convert4/1
  reg2/1 -> Convert3/1
  reg3/1 -> Convert2/1
  reg1/1 -> Convert1/1
  reg9/1 -> Convert/1
  din4/1 -> reg7/1
  din7/1 -> reg5/1
  din6/1 -> reg6/1
  din5/1 -> reg4/1
  din3/1 -> reg2/1
  din2/1 -> reg3/1
  din1/1 -> reg1/1
  trig/1 -> [trig]
  we/1 -> [we]
  din0/1 -> reg9/1

== system amila/feng0_coarse_delay ==
  sim_1 : Inport
  amila_feng0_coarse_delay_user_data_out : xbsIndex_r4/Gateway In  gui_display_data_type=Fixed-point  arith_type=Unsigned  n_bits=32  bin_pt=0  preci_type=Single  exp_width=8  frac_width=24  quantization="Round  (unbiased: +/- Inf)"  overflow=Saturate  period=1  dbl_ovrd=off  timing_constraint=None  locs_specified=off  LOCs={}  UseAsADC=off  ADCChannel='1'  inherit_from_input=off  hdl_port=on  block_type=gatewayin
  io_delay : xbsIndex_r4/Delay  rst=off  infoeditControl=Selection of Reset will increase slice count due to use of real FFs and instead of SRLs  en=off  latency=0  dbl_ovrd=off  reg_retiming=on  block_type=delay
  reint1 : xbsIndex_r4/Reinterpret  force_arith_type=on  arith_type=Unsigned  force_bin_pt=on  bin_pt=0  block_type=reinterpret
  slice_reg : xbsIndex_r4/Slice  nbits=32  boolean_output=off  mode=Lower Bit Location + Width  bit1=0  base1=MSB of Input  bit0=0  base0=LSB of Input  dbl_ovrd=off  block_type=slice
  in_reg : Outport
  wires:
  amila_feng0_coarse_delay_user_data_out/1 -> io_delay/1
  sim_1/1 -> amila_feng0_coarse_delay_user_data_out/1
  io_delay/1 -> slice_reg/1
  slice_reg/1 -> reint1/1
  reint1/1 -> in_reg/1

== system amila/feng0_ctrl ==
  sim_1 : Inport
  amila_feng0_ctrl_user_data_out : xbsIndex_r4/Gateway In  gui_display_data_type=Fixed-point  arith_type=Unsigned  n_bits=32  bin_pt=0  preci_type=Single  exp_width=8  frac_width=24  quantization="Round  (unbiased: +/- Inf)"  overflow=Saturate  period=1  dbl_ovrd=off  timing_constraint=None  locs_specified=off  LOCs={}  UseAsADC=off  ADCChannel='1'  inherit_from_input=off  hdl_port=on  block_type=gatewayin
  io_delay : xbsIndex_r4/Delay  rst=off  infoeditControl=Selection of Reset will increase slice count due to use of real FFs and instead of SRLs  en=off  latency=0  dbl_ovrd=off  reg_retiming=on  block_type=delay
  reint1 : xbsIndex_r4/Reinterpret  force_arith_type=on  arith_type=Unsigned  force_bin_pt=on  bin_pt=0  block_type=reinterpret
  slice_reg : xbsIndex_r4/Slice  nbits=32  boolean_output=off  mode=Lower Bit Location + Width  bit1=0  base1=MSB of Input  bit0=0  base0=LSB of Input  dbl_ovrd=off  block_type=slice
  in_reg : Outport
  wires:
  amila_feng0_ctrl_user_data_out/1 -> io_delay/1
  sim_1/1 -> amila_feng0_ctrl_user_data_out/1
  io_delay/1 -> slice_reg/1
  slice_reg/1 -> reint1/1
  reint1/1 -> in_reg/1
